simulink model "drone"  (R2024b)
settings: Solver=VariableStepAuto  StartTime=0.0  StopTime=10.0  RelTol=1e-3
values from neighbouring files (symbols this model uses):
  controlador = projetarControladorDrone(requisitos, planta)    [executarAnaliseFiltros.m]
  modo = MODO_FILTRO    (= 3)    [executarAnaliseFiltros.m]
  planta = obterPlantaDrone()    [executarAnaliseFiltros.m]
  varz = varzs(i)    [executarAnaliseFiltros.m]
undefined symbols (not defined in the file or in its folder): referencia, sensor
settings Model: Creator=brunn  LastModifiedBy=brunn

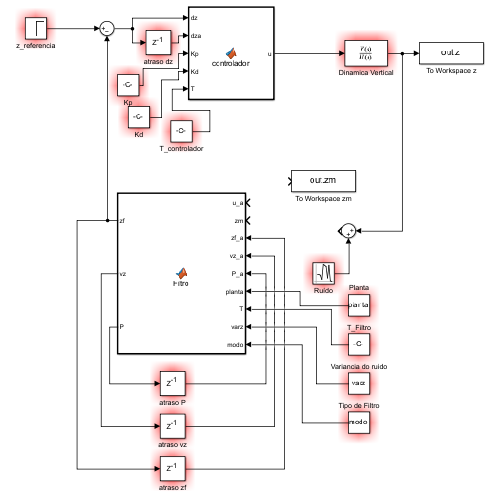
[thumbnail: Simulink's stored preview of the top-level diagram]
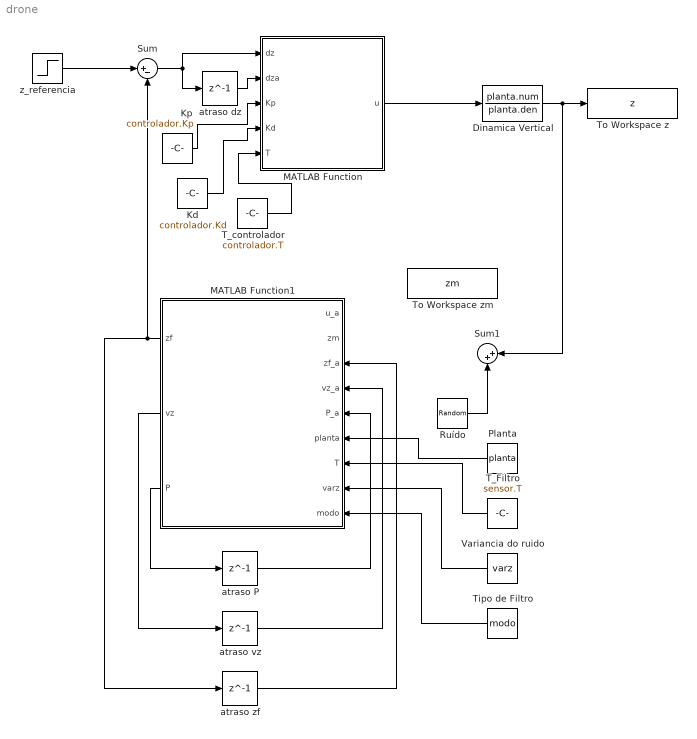
== system drone ==
  Dinamica Vertical : TransferFcn  Numerator=planta.num  Denominator=planta.den
  Kd : Constant  Value=controlador.Kd
  Kp : Constant  Value=controlador.Kp
  MATLAB Function : MATLAB Function  TreatAsAtomicUnit=on
  MATLAB Function1 : MATLAB Function  TreatAsAtomicUnit=on
  Planta : Constant  Value=planta
  "Ruído " : RandomNumber  Variance=varz  SampleTime=sensor.T
  Sum : Sum  Inputs=|+-
  Sum1 : Sum  Inputs=|++
  T_Filtro : Constant  Value=sensor.T
  T_controlador : Constant  Value=controlador.T
  Tipo de Filtro : Constant  Value=modo
  To Workspace z : ToWorkspace  VariableName=z  SaveFormat=Timeseries  SampleTime=-1
  To Workspace zm : ToWorkspace  VariableName=zm  SaveFormat=Timeseries  SampleTime=-1
  Variancia do ruido : Constant  Value=varz
  atraso P : Delay  DelayLength=1  InitialCondition=0  SampleTime=sensor.T
  atraso dz : Delay  DelayLength=1  InitialCondition=0  SampleTime=controlador.T
  atraso vz : Delay  DelayLength=1  InitialCondition=0  SampleTime=sensor.T
  atraso zf : Delay  DelayLength=1  InitialCondition=0  SampleTime=sensor.T
  z_referencia : Step  Time=referencia.instante  After=referencia.amplitude  SampleTime=0
  wires:
  z_referencia/1 -> Sum/1
  Sum/1 -> atraso dz/1, MATLAB Function/1(dz)
  MATLAB Function/1(u) -> Dinamica Vertical/1
  Dinamica Vertical/1 -> To Workspace z/1, Sum1/1
  "Ruído "/1 -> Sum1/2
  T_controlador/1 -> MATLAB Function/5(T)
  atraso dz/1 -> MATLAB Function/2(dza)
  Kp/1 -> MATLAB Function/3(Kp)
  Kd/1 -> MATLAB Function/4(Kd)
  MATLAB Function1/2(vz) -> atraso vz/1
  MATLAB Function1/3(P) -> atraso P/1
  MATLAB Function1/1(zf) -> atraso zf/1, Sum/2
  atraso zf/1 -> MATLAB Function1/3(zf_a)
  atraso vz/1 -> MATLAB Function1/4(vz_a)
  atraso P/1 -> MATLAB Function1/5(P_a)
  T_Filtro/1 -> MATLAB Function1/7(T)
  Variancia do ruido/1 -> MATLAB Function1/8(varz)
  Tipo de Filtro/1 -> MATLAB Function1/9(modo)
  Planta/1 -> MATLAB Function1/6(planta)

== matlab function drone/MATLAB Function1 ==
  data: zf output; u_a input; zm input; zf_a input; vz_a input; P_a input; planta input; T input; varz input; modo input; vz output; P output
function [zf, vz, P] = Filtro(u_a, zm, zf_a, vz_a, P_a, planta, T, varz, modo)

if modo==1 % sem filtro
    zf = zm;
    vz = 0;
    P = eye(2);
end

if modo==2 % filtro passa-baixa
    alpha = 0.73;
    zf = alpha * zf_a + (1 - alpha) * zm;
    vz = 0;
    P = eye(2);
end

if modo==3 % filtro Kalman
    if zf==0
        P_a = eye(2);
    end

    F = [1 T; 0 1-T*planta.b/planta.m];
    G = [0.5*T^2/planta.m; T/modo];
    H = [1 0];
    
    Q = [0.0001 0; 0 0.001];
    
    R = varz;

    estado_novo = F * [zf_a; vz_a] + G * u_a;
    P_novo = F * P_a * F' + Q;

    K = P_novo * H' / (H * P_novo * H' + R);

    estado = estado_novo + K * (zm - H * estado_novo);
    
    P = (eye(2) - K * H) * P_novo;

    zf = estado(1);
    vz = estado(2);

end

== matlab function drone/MATLAB Function ==
  data: dz input; u output; dza input; Kp input; Kd input; T input
function u = controlador(dz, dza, Kp, Kd, T)

u = Kp*dz + Kd*(dz-dza)/T;
